simulink model "N_WS"  (R2024b)
settings: Solver=VariableStepAuto  StartTime=0.0  StopTime=10.0  RelTol=1e-3
values from neighbouring files (symbols this model uses):
  Ga = 0.112    [P7.m]
  Gf = 1/(Gs*Kd)    (= 0.25)    [P7.m]
  Gs = 0.5    [P7.m]
libraries: cstblocks x2
settings Model: Creator=lucap  LastModifiedBy=lucap

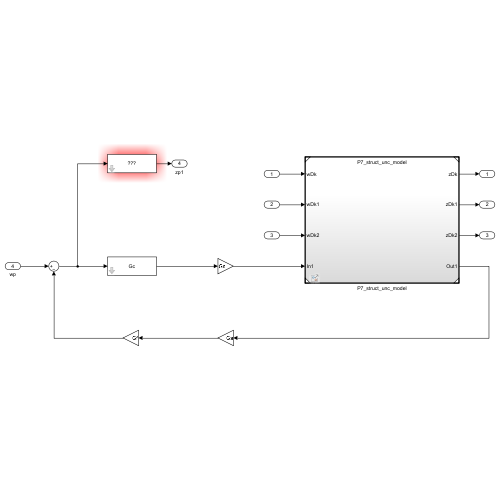
[thumbnail: Simulink's stored preview of the top-level diagram]
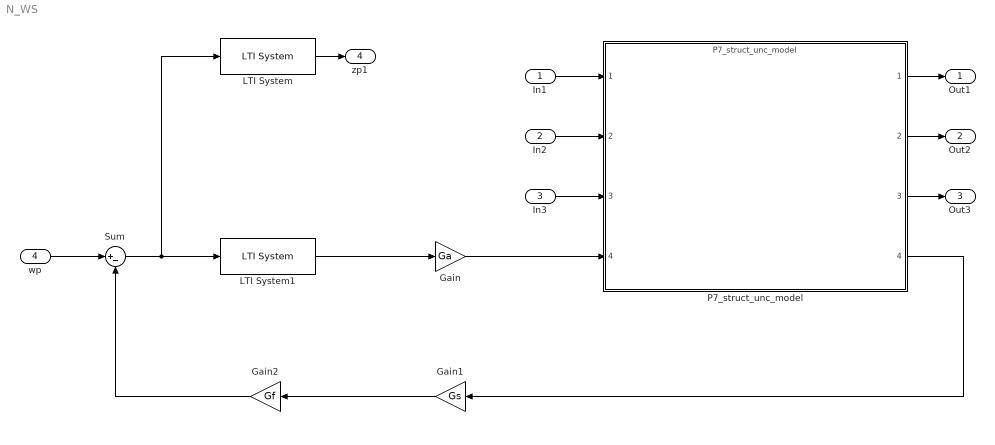
== system N_WS ==
  In1 : Inport
  In2 : Inport  Port=2
  In3 : Inport  Port=3
  wp : Inport  Port=4
  Gain : Gain  Gain=Ga
  Gain1 : Gain  Gain=Gs
  Gain2 : Gain  Gain=Gf
  LTI System : cstblocks/LTI System  sys=Ws_mu  IC=[]  PadeOrder=0
  LTI System1 : cstblocks/LTI System  sys=Gc  IC=[]  PadeOrder=0
  P7_struct_unc_model : ModelReference  ModelNameDialog=P7_struct_unc_model.slx  SimulationMode=Normal  ModelReferenceVersion=1.1
  Sum : Sum  Inputs=|+-
  Out1 : Outport
  Out2 : Outport  Port=2
  Out3 : Outport  Port=3
  zp1 : Outport  Port=4
  wires:
  In1/1 -> P7_struct_unc_model/1
  In2/1 -> P7_struct_unc_model/2
  In3/1 -> P7_struct_unc_model/3
  P7_struct_unc_model/1 -> Out1/1
  P7_struct_unc_model/2 -> Out2/1
  P7_struct_unc_model/3 -> Out3/1
  LTI System1/1 -> Gain/1
  Gain/1 -> P7_struct_unc_model/4
  Gain1/1 -> Gain2/1
  wp/1 -> Sum/1
  LTI System/1 -> zp1/1
  Sum/1 -> LTI System/1, LTI System1/1
  Gain2/1 -> Sum/2
  P7_struct_unc_model/4 -> Gain1/1
